simulink subsystem "Linear_Generator_AC_DC_Converter_SS"  (R2021b)
settings: Solver=VariableStepAuto  StartTime=0.0  StopTime=10.0  RelTol=1e-3
model mask{ptoSim=ptoSim.directLinearGenerator(1)}
  mask prompts: ptoSim "Machine Name"
undefined symbols (not defined in the file): absPower, elecPower, force, fricForce, Ia, Ib, Ic, simu, Va, Vb, Vc, vel
settings Model: Creator=Derek  LastModifiedBy=Derek

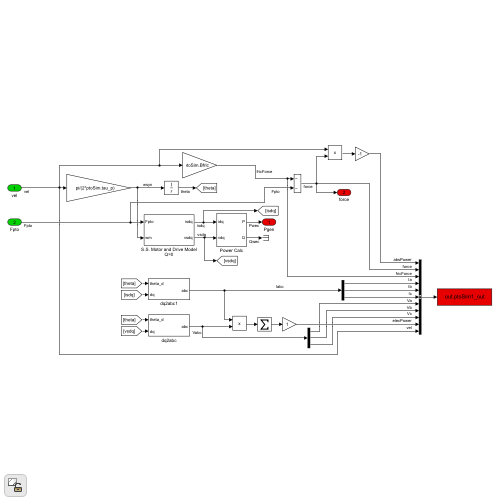
[thumbnail: Simulink's stored preview of the top-level diagram]
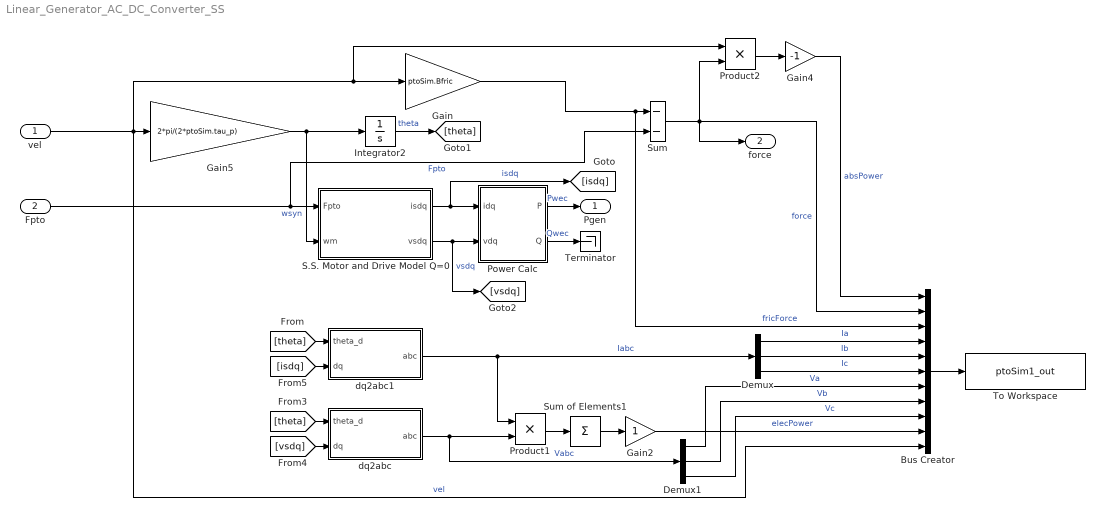
== system Linear_Generator_AC_DC_Converter_SS ==
  vel : Inport
  Fpto : Inport  Port=2
  Bus Creator : BusCreator  Inputs=absPower,force,fricForce,Ia,Ib,Ic,Va,Vb,Vc,elecPower,vel
  Demux : Demux  Outputs=3
  Demux1 : Demux  Outputs=3
  Gain : Gain  Gain=ptoSim.Bfric
  Gain2 : Gain
  Gain4 : Gain  Gain=-1
  Gain5 : Gain  Gain=2*pi/(2*ptoSim.tau_p)
  Integrator2 : Integrator  InitialCondition=ptoSim.theta_d_0
  Power Calc : Subsystem
  Product1 : Product
  Product2 : Product
  S.S. Motor and Drive Model Q=0 : Subsystem
  Sum : Sum  Inputs=--
  Sum of Elements1 : Sum  Inputs=+
  Terminator : Terminator
  To Workspace : ToWorkspace  VariableName=ptoSim1_out  SaveFormat=Structure With Time  SampleTime=simu.dtOut
  dq2abc : Subsystem
  dq2abc1 : Subsystem
  Pgen : Outport
  force : Outport  Port=2
  wires:
  Gain/1 -> Bus Creator/3, Sum/1  "fricForce"
  S.S. Motor and Drive Model Q=0/2(vsdq) -> Power Calc/2(vdq), [vsdq]  "vsdq"
  Sum/1 -> Bus Creator/2, force/1, Product2/2  "force"
  Sum of Elements1/1 -> Gain2/1
  Integrator2/1 -> [theta]  "theta"
  vel/1 -> Gain5/1, Bus Creator/11, Product2/1, Gain/1  "vel"
  Gain2/1 -> Bus Creator/10  "elecPower"
  Product1/1 -> Sum of Elements1/1
  dq2abc/1(abc) -> Product1/2, Demux1/1  "Vabc"
  Demux1/3 -> Bus Creator/9  "Vc"
  Demux1/2 -> Bus Creator/8  "Vb"
  Demux/3 -> Bus Creator/6  "Ic"
  Gain5/1 -> S.S. Motor and Drive Model Q=0/2(wm), Integrator2/1  "wsyn"
  Demux1/1 -> Bus Creator/7  "Va"
  Demux/1 -> Bus Creator/4  "Ia"
  S.S. Motor and Drive Model Q=0/1(isdq) -> [isdq], Power Calc/1(idq)  "isdq"
  Bus Creator/1 -> To Workspace/1
  Demux/2 -> Bus Creator/5  "Ib"
  dq2abc1/1(abc) -> Demux/1, Product1/1  "Iabc"
  Gain4/1 -> Bus Creator/1  "absPower"
  Product2/1 -> Gain4/1
  Power Calc/2(Q) -> Terminator/1  "Qwec"
  Power Calc/1(P) -> Pgen/1  "Pwec"
  [theta] -> dq2abc1/1(theta_d)
  [theta] -> dq2abc/1(theta_d)
  [vsdq] -> dq2abc/2(dq)
  [isdq] -> dq2abc1/2(dq)
  Fpto/1 -> Sum/2, S.S. Motor and Drive Model Q=0/1(Fpto)  "Fpto"

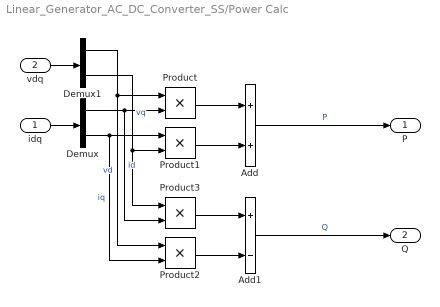
== system Linear_Generator_AC_DC_Converter_SS/Power Calc ==
  idq : Inport
  vdq : Inport  Port=2
  Add : Sum
  Add1 : Sum  Inputs=+-
  Demux : Demux  Outputs=2
  Demux1 : Demux  Outputs=2
  Product{,1..3} (4 alike) : Product
  P : Outport
  Q : Outport  Port=2
  wires:
  vdq/1 -> Demux1/1
  idq/1 -> Demux/1
  Add/1 -> P/1  "P"
  Product/1 -> Add/1
  Product2/1 -> Add1/2
  Product3/1 -> Add1/1
  Demux/2 -> Product1/1, Product2/2  "iq"
  Demux1/1 -> Product2/1, Product/1  "vd"
  Demux1/2 -> Product3/1, Product1/2  "vq"
  Add1/1 -> Q/1  "Q"
  Product1/1 -> Add/2
  Demux/1 -> Product/2, Product3/2  "id"

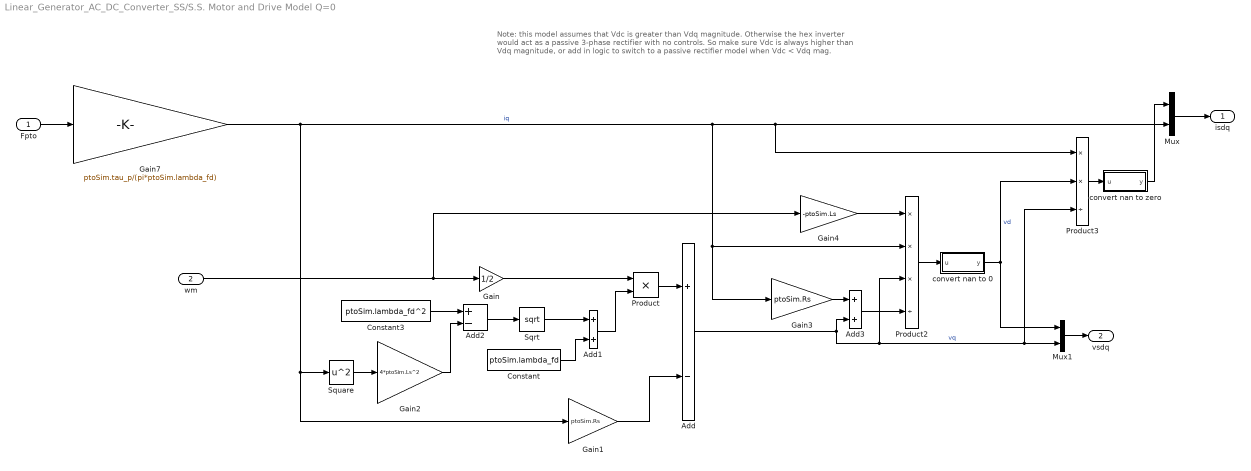
== system Linear_Generator_AC_DC_Converter_SS/S.S. Motor and Drive Model Q=0 ==
  note: Note: this model assumes that Vdc is greater than Vdq magnitude. Otherwise the hex inverter would act as a passive 3-phase rectifier with no controls. So make sure Vdc is always higher than Vdq magnitude, or add in logic to switch to a passive rectifier model when Vdc < Vdq mag.
  Fpto : Inport
  wm : Inport  Port=2
  Add : Sum  Inputs=+-
  Add1 : Sum
  Add2 : Sum  Inputs=+-
  Add3 : Sum
  Constant : Constant  Value=ptoSim.lambda_fd
  Constant3 : Constant  Value=ptoSim.lambda_fd^2
  Gain : Gain  Gain=1/2
  Gain1 : Gain  Gain=ptoSim.Rs
  Gain2 : Gain  Gain=4*ptoSim.Ls^2
  Gain3 : Gain  Gain=ptoSim.Rs
  Gain4 : Gain  Gain=-ptoSim.Ls
  Gain7 : Gain  Gain=ptoSim.tau_p/(pi*ptoSim.lambda_fd)
  Mux : Mux  Inputs=2
  Mux1 : Mux  Inputs=2
  Product : Product
  Product2 : Product  Inputs=***/
  Product3 : Product  Inputs=**/
  Sqrt : Sqrt  SaturateOnIntegerOverflow=on
  Square : Math  Operator=square  SaturateOnIntegerOverflow=on
  convert nan to 0 : MATLAB Function  TreatAsAtomicUnit=on
  convert nan to zero : MATLAB Function  TreatAsAtomicUnit=on
  isdq : Outport
  vsdq : Outport  Port=2
  wires:
  wm/1 -> Gain/1, Gain4/1
  Square/1 -> Gain2/1
  Product3/1 -> convert nan to zero/1(u)
  Gain4/1 -> Product2/1
  Gain3/1 -> Add3/1
  Add3/1 -> Product2/4
  Product2/1 -> convert nan to 0/1(u)
  Gain2/1 -> Add2/2
  Constant3/1 -> Add2/1
  Add2/1 -> Sqrt/1
  Sqrt/1 -> Add1/1
  Add1/1 -> Product/2
  Gain/1 -> Product/1
  Product/1 -> Add/1
  Gain1/1 -> Add/2
  convert nan to zero/1(y) -> Mux/1
  Add/1 -> Add3/2, Mux1/2, Product3/3, Product2/3  "vq"
  convert nan to 0/1(y) -> Mux1/1, Product3/2  "vd"
  Constant/1 -> Add1/2
  Gain7/1 -> Square/1, Gain1/1, Mux/2, Product3/1, Gain3/1, Product2/2  "iq"
  Mux1/1 -> vsdq/1
  Mux/1 -> isdq/1
  Fpto/1 -> Gain7/1

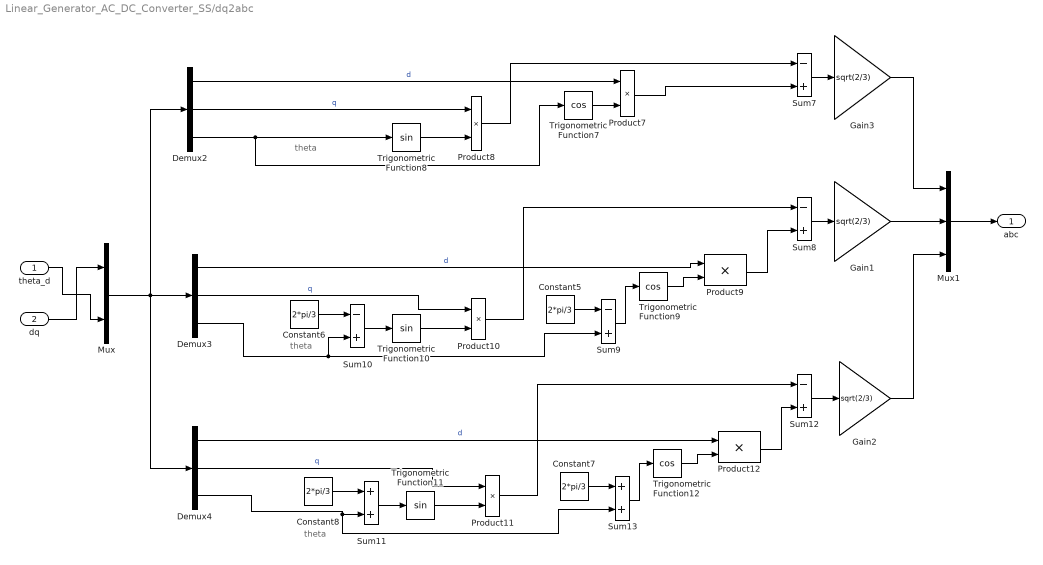
== system Linear_Generator_AC_DC_Converter_SS/dq2abc ==
  note: theta
  note: theta
  note: theta
  theta_d : Inport
  dq : Inport  Port=2
  Constant{5..8} (4 alike) : Constant  Value=2*pi/3
  Demux2 : Demux  Outputs=3
      settings: DisplayOption=none
  Demux3 : Demux  Outputs=3
      settings: DisplayOption=none
  Demux4 : Demux  Outputs=3
      settings: DisplayOption=none
  Gain1 : Gain  Gain=sqrt(2/3)  SaturateOnIntegerOverflow=on  OutDataTypeStr=Inherit: Same as input  ParamDataTypeStr=Inherit: Same as input
  Gain2 : Gain  Gain=sqrt(2/3)  SaturateOnIntegerOverflow=on  OutDataTypeStr=Inherit: Same as input  ParamDataTypeStr=Inherit: Same as input
  Gain3 : Gain  Gain=sqrt(2/3)  SaturateOnIntegerOverflow=on  OutDataTypeStr=Inherit: Same as input  ParamDataTypeStr=Inherit: Same as input
  Mux : Mux  Inputs=2
  Mux1 : Mux  Inputs=3
  Product{7..12} (6 alike) : Product  InputSameDT=on  SaturateOnIntegerOverflow=on  OutDataTypeStr=Inherit: Same as first input
  Sum{7..10,12} (5 alike) : Sum  Inputs=-+  InputSameDT=on  SaturateOnIntegerOverflow=on  OutDataTypeStr=Inherit: Same as first input
  Sum11 : Sum  InputSameDT=on  SaturateOnIntegerOverflow=on  OutDataTypeStr=Inherit: Same as first input
  Sum13 : Sum  InputSameDT=on  SaturateOnIntegerOverflow=on  OutDataTypeStr=Inherit: Same as first input
  Trigonometric Function10 : Trigonometry
  Trigonometric Function11 : Trigonometry
  Trigonometric Function12 : Trigonometry  Operator=cos
  Trigonometric Function7 : Trigonometry  Operator=cos
  Trigonometric Function8 : Trigonometry
  Trigonometric Function9 : Trigonometry  Operator=cos
  abc : Outport
  wires:
  Constant7/1 -> Sum13/1
  Trigonometric Function11/1 -> Product11/2
  Trigonometric Function8/1 -> Product8/2
  Demux3/1 -> Product9/1  "d"
  Sum9/1 -> Trigonometric Function9/1
  Sum8/1 -> Gain1/1
  Trigonometric Function9/1 -> Product9/2
  Sum11/1 -> Trigonometric Function11/1
  theta_d/1 -> Mux/2
  Sum12/1 -> Gain2/1
  Mux/1 -> Demux4/1, Demux2/1, Demux3/1
  Gain3/1 -> Mux1/1
  Sum10/1 -> Trigonometric Function10/1
  Demux2/1 -> Product7/1  "d"
  Demux4/3 -> Sum13/2, Sum11/2
  Gain2/1 -> Mux1/3
  Demux4/1 -> Product12/1  "d"
  Trigonometric Function10/1 -> Product10/2
  Trigonometric Function12/1 -> Product12/2
  Constant5/1 -> Sum9/1
  Trigonometric Function7/1 -> Product7/2
  dq/1 -> Mux/1
  Demux2/2 -> Product8/1  "q"
  Demux3/2 -> Product10/1  "q"
  Demux3/3 -> Sum10/2, Sum9/2
  Mux1/1 -> abc/1
  Product8/1 -> Sum7/1
  Constant6/1 -> Sum10/1
  Product12/1 -> Sum12/2
  Demux2/3 -> Trigonometric Function8/1, Trigonometric Function7/1
  Sum13/1 -> Trigonometric Function12/1
  Product11/1 -> Sum12/1
  Product10/1 -> Sum8/1
  Demux4/2 -> Product11/1  "q"
  Sum7/1 -> Gain3/1
  Product9/1 -> Sum8/2
  Gain1/1 -> Mux1/2
  Product7/1 -> Sum7/2
  Constant8/1 -> Sum11/1

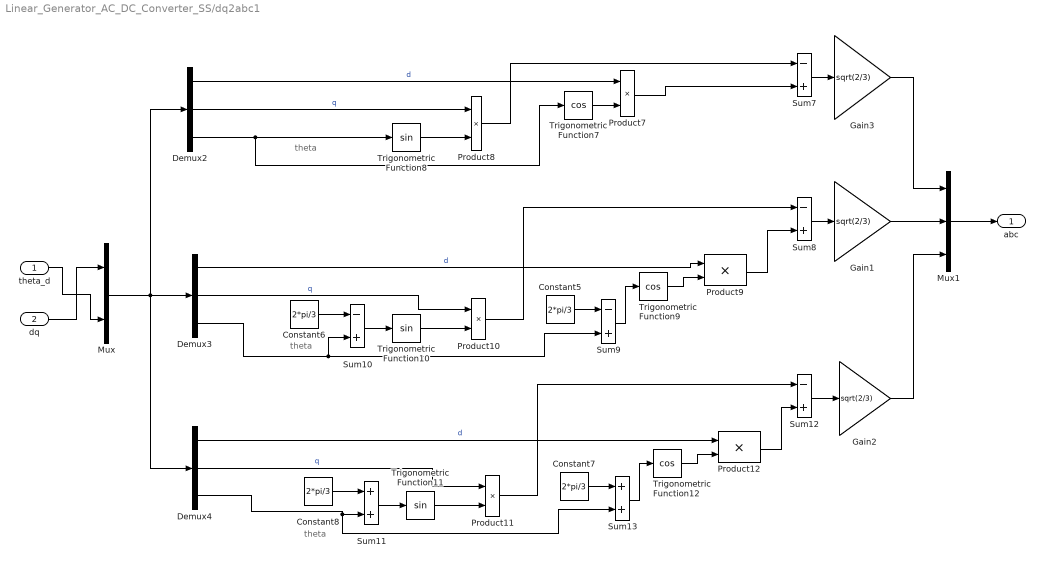
== system Linear_Generator_AC_DC_Converter_SS/dq2abc1 ==
  note: theta
  note: theta
  note: theta
  theta_d : Inport
  dq : Inport  Port=2
  Constant{5..8} (4 alike) : Constant  Value=2*pi/3
  Demux2 : Demux  Outputs=3
      settings: DisplayOption=none
  Demux3 : Demux  Outputs=3
      settings: DisplayOption=none
  Demux4 : Demux  Outputs=3
      settings: DisplayOption=none
  Gain1 : Gain  Gain=sqrt(2/3)  SaturateOnIntegerOverflow=on  OutDataTypeStr=Inherit: Same as input  ParamDataTypeStr=Inherit: Same as input
  Gain2 : Gain  Gain=sqrt(2/3)  SaturateOnIntegerOverflow=on  OutDataTypeStr=Inherit: Same as input  ParamDataTypeStr=Inherit: Same as input
  Gain3 : Gain  Gain=sqrt(2/3)  SaturateOnIntegerOverflow=on  OutDataTypeStr=Inherit: Same as input  ParamDataTypeStr=Inherit: Same as input
  Mux : Mux  Inputs=2
  Mux1 : Mux  Inputs=3
  Product{7..12} (6 alike) : Product  InputSameDT=on  SaturateOnIntegerOverflow=on  OutDataTypeStr=Inherit: Same as first input
  Sum{7..10,12} (5 alike) : Sum  Inputs=-+  InputSameDT=on  SaturateOnIntegerOverflow=on  OutDataTypeStr=Inherit: Same as first input
  Sum11 : Sum  InputSameDT=on  SaturateOnIntegerOverflow=on  OutDataTypeStr=Inherit: Same as first input
  Sum13 : Sum  InputSameDT=on  SaturateOnIntegerOverflow=on  OutDataTypeStr=Inherit: Same as first input
  Trigonometric Function10 : Trigonometry
  Trigonometric Function11 : Trigonometry
  Trigonometric Function12 : Trigonometry  Operator=cos
  Trigonometric Function7 : Trigonometry  Operator=cos
  Trigonometric Function8 : Trigonometry
  Trigonometric Function9 : Trigonometry  Operator=cos
  abc : Outport
  wires:
  Constant7/1 -> Sum13/1
  Trigonometric Function11/1 -> Product11/2
  Trigonometric Function8/1 -> Product8/2
  Demux3/1 -> Product9/1  "d"
  Sum9/1 -> Trigonometric Function9/1
  Sum8/1 -> Gain1/1
  Trigonometric Function9/1 -> Product9/2
  Sum11/1 -> Trigonometric Function11/1
  theta_d/1 -> Mux/2
  Sum12/1 -> Gain2/1
  Mux/1 -> Demux4/1, Demux2/1, Demux3/1
  Gain3/1 -> Mux1/1
  Sum10/1 -> Trigonometric Function10/1
  Demux2/1 -> Product7/1  "d"
  Demux4/3 -> Sum13/2, Sum11/2
  Gain2/1 -> Mux1/3
  Demux4/1 -> Product12/1  "d"
  Trigonometric Function10/1 -> Product10/2
  Trigonometric Function12/1 -> Product12/2
  Constant5/1 -> Sum9/1
  Trigonometric Function7/1 -> Product7/2
  dq/1 -> Mux/1
  Demux2/2 -> Product8/1  "q"
  Demux3/2 -> Product10/1  "q"
  Demux3/3 -> Sum10/2, Sum9/2
  Mux1/1 -> abc/1
  Product8/1 -> Sum7/1
  Constant6/1 -> Sum10/1
  Product12/1 -> Sum12/2
  Demux2/3 -> Trigonometric Function8/1, Trigonometric Function7/1
  Sum13/1 -> Trigonometric Function12/1
  Product11/1 -> Sum12/1
  Product10/1 -> Sum8/1
  Demux4/2 -> Product11/1  "q"
  Sum7/1 -> Gain3/1
  Product9/1 -> Sum8/2
  Gain1/1 -> Mux1/2
  Product7/1 -> Sum7/2
  Constant8/1 -> Sum11/1

== matlab function Linear_Generator_AC_DC_Converter_SS/S.S. Motor and Drive Model Q=0/convert nan to zero ==
  data: u input; y output
function y = fcn(u)
if isnan(u)
    y=0;
else
    y = u;
end
end

== matlab function Linear_Generator_AC_DC_Converter_SS/S.S. Motor and Drive Model Q=0/convert nan to 0 ==
  data: u input; y output
function y = fcn(u)
if isnan(u)
    y=0;
else
    y = u;
end
end
